simulink model "ex_4_PID"  (R2018a)
settings: Solver=VariableStepAuto  StartTime=0.0  StopTime=20  RelTol=1e-3
values from neighbouring files (symbols this model uses):
  b = 1    [EX4_MATHLAB_SCRIPT.m]
  D = 5    [EX4_MATHLAB_SCRIPT.m]
  den1 = [J*Ra,Kb*Km,K*Km]    [EX4_MATHLAB_SCRIPT.m]
  den2 = [J*Ra,Kb*Km,K*Km]    [EX4_MATHLAB_SCRIPT.m]
  I = 10    [EX4_MATHLAB_SCRIPT.m]
  J = 0.1    [EX4_MATHLAB_SCRIPT.m]
  Kb = 1    [EX4_MATHLAB_SCRIPT.m]
  Km = 0.1    [EX4_MATHLAB_SCRIPT.m]
  La = 1    [EX4_MATHLAB_SCRIPT.m]
  n = 10    [EX4_MATHLAB_SCRIPT.m]
  num1 = [K*Km]    [EX4_MATHLAB_SCRIPT.m]
  num2 = [Km,0]    [EX4_MATHLAB_SCRIPT.m]
  P = 50    [EX4_MATHLAB_SCRIPT.m]
  Ra = 20    [EX4_MATHLAB_SCRIPT.m]
libraries: simulink x2
settings Model: Creator=k2202936  LastModifiedBy=k2202936

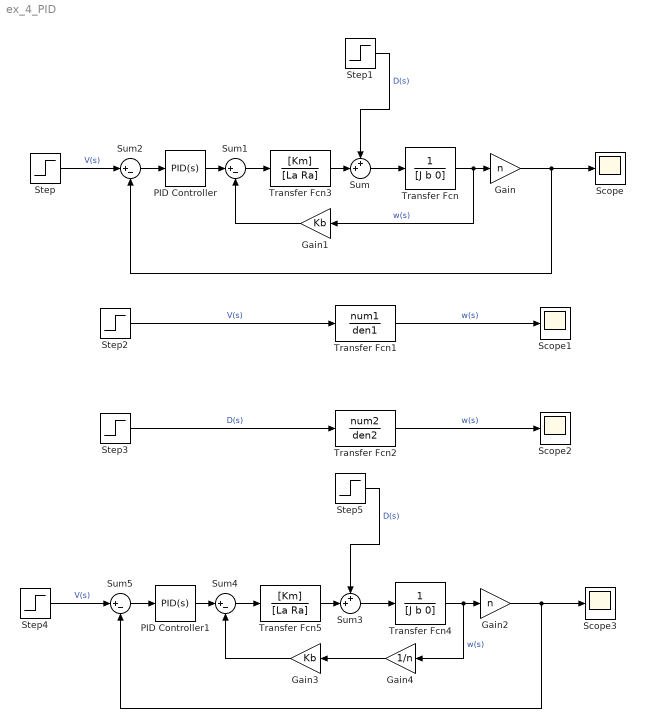
== system ex_4_PID ==
  Gain : Gain  Gain=n
  Gain1 : Gain  Gain=Kb
  Gain2 : Gain  Gain=n
  Gain3 : Gain  Gain=Kb
  Gain4 : Gain  Gain=1/n
  PID Controller : simulink/Continuous/PID Controller  Controller=PID  TimeDomain=Continuous-time  SampleTime=-1  IntegratorMethod=Forward Euler  FilterMethod=Forward Euler  Form=Parallel  UseFilter=on  ControllerParametersSource=internal  P=P  I=I  D=D  N=100  InitialConditionSource=internal  InitialConditionForIntegrator=0  InitialConditionForFilter=0  ExternalReset=none  LimitOutput=off  UpperSaturationLimit=inf  LowerSaturationLimit=-inf  LinearizeAsGain=on  AntiWindupMode=none  Kb=1  TrackingMode=off  Kt=1  PParamMin=[]  PParamMax=[]  IParamMin=[]  IParamMax=[]  DParamMin=[]  DParamMax=[]  NParamMin=[]  NParamMax=[]  KbParamMin=[]  KbParamMax=[]  KtParamMin=[]  KtParamMax=[]  POutMin=[]  POutMax=[]  IOutMin=[]  IOutMax=[]  DOutMin=[]  DOutMax=[]  NOutMin=[]  NOutMax=[]  KbOutMin=[]  KbOutMax=[]  KtOutMin=[]  KtOutMax=[]  IntegratorOutMin=[]  IntegratorOutMax=[]  FilterOutMin=[]  FilterOutMax=[]  SumOutMin=[]  SumOutMax=[]  SumI1OutMin=[]  SumI1OutMax=[]  SumI2OutMin=[]  SumI2OutMax=[]  SumI3OutMin=[]  SumI3OutMax=[]  SumDOutMin=[]  SumDOutMax=[]  SaturationOutMin=[]  SaturationOutMax=[]  IntegratorContinuousStateAttributes=''  IntegratorStateMustResolveToSignalObject=off  IntegratorRTWStateStorageClass=Auto  FilterContinuousStateAttributes=''  FilterStateMustResolveToSignalObject=off  FilterRTWStateStorageClass=Auto  DifferentiatorICPrevScaledInput=0  DifferentiatorOutMin=[]  DifferentiatorOutMax=[]  FilterDiffOutCoefMin=[]  FilterDiffOutCoefMax=[]  SumDenOutMin=[]  SumDenOutMax=[]  SumNumOutMin=[]  SumNumOutMax=[]  ReciprocalOutMin=[]  ReciprocalOutMax=[]  DivideOutMin=[]  DivideOutMax=[]  TunerSelectOption=Transfer Function Based (PID Tuner App)
  PID Controller1 : simulink/Continuous/PID Controller  Controller=PID  TimeDomain=Continuous-time  SampleTime=-1  IntegratorMethod=Forward Euler  FilterMethod=Forward Euler  Form=Parallel  UseFilter=on  ControllerParametersSource=internal  P=P  I=I  D=D  N=100  InitialConditionSource=internal  InitialConditionForIntegrator=0  InitialConditionForFilter=0  ExternalReset=none  LimitOutput=off  UpperSaturationLimit=inf  LowerSaturationLimit=-inf  LinearizeAsGain=on  AntiWindupMode=none  Kb=1  TrackingMode=off  Kt=1  PParamMin=[]  PParamMax=[]  IParamMin=[]  IParamMax=[]  DParamMin=[]  DParamMax=[]  NParamMin=[]  NParamMax=[]  KbParamMin=[]  KbParamMax=[]  KtParamMin=[]  KtParamMax=[]  POutMin=[]  POutMax=[]  IOutMin=[]  IOutMax=[]  DOutMin=[]  DOutMax=[]  NOutMin=[]  NOutMax=[]  KbOutMin=[]  KbOutMax=[]  KtOutMin=[]  KtOutMax=[]  IntegratorOutMin=[]  IntegratorOutMax=[]  FilterOutMin=[]  FilterOutMax=[]  SumOutMin=[]  SumOutMax=[]  SumI1OutMin=[]  SumI1OutMax=[]  SumI2OutMin=[]  SumI2OutMax=[]  SumI3OutMin=[]  SumI3OutMax=[]  SumDOutMin=[]  SumDOutMax=[]  SaturationOutMin=[]  SaturationOutMax=[]  IntegratorContinuousStateAttributes=''  IntegratorStateMustResolveToSignalObject=off  IntegratorRTWStateStorageClass=Auto  FilterContinuousStateAttributes=''  FilterStateMustResolveToSignalObject=off  FilterRTWStateStorageClass=Auto  DifferentiatorICPrevScaledInput=0  DifferentiatorOutMin=[]  DifferentiatorOutMax=[]  FilterDiffOutCoefMin=[]  FilterDiffOutCoefMax=[]  SumDenOutMin=[]  SumDenOutMax=[]  SumNumOutMin=[]  SumNumOutMax=[]  ReciprocalOutMin=[]  ReciprocalOutMax=[]  DivideOutMin=[]  DivideOutMax=[]  TunerSelectOption=Transfer Function Based (PID Tuner App)
  Scope{,1..3} (4 alike) : Scope
  Step{,2..3,5} (4 alike) : Step  Time=0  SampleTime=0
  Step1 : Step  Time=0  After=0  SampleTime=0
  Step4 : Step  Time=0  After=0  SampleTime=0
  Sum : Sum  Inputs=++|
  Sum{1..2,4..5} (4 alike) : Sum  Inputs=|+-
  Sum3 : Sum  Inputs=++|
  Transfer Fcn : TransferFcn  Denominator=[J b 0]
  Transfer Fcn1 : TransferFcn  Numerator=num1  Denominator=den1
  Transfer Fcn2 : TransferFcn  Numerator=num2  Denominator=den2
  Transfer Fcn3 : TransferFcn  Numerator=[Km]  Denominator=[La Ra]
  Transfer Fcn4 : TransferFcn  Denominator=[J b 0]
  Transfer Fcn5 : TransferFcn  Numerator=[Km]  Denominator=[La Ra]
  wires:
  Step3/1 -> Transfer Fcn2/1  "D(s)"
  Step2/1 -> Transfer Fcn1/1  "V(s)"
  Transfer Fcn2/1 -> Scope2/1  "w(s)"
  Transfer Fcn1/1 -> Scope1/1  "w(s)"
  Sum/1 -> Transfer Fcn/1
  Sum2/1 -> PID Controller/1
  Transfer Fcn/1 -> Gain1/1, Gain/1  "w(s)"
  Sum1/1 -> Transfer Fcn3/1
  Step/1 -> Sum2/1  "V(s)"
  Transfer Fcn3/1 -> Sum/2
  Step1/1 -> Sum/1  "D(s)"
  PID Controller/1 -> Sum1/1
  Gain1/1 -> Sum1/2
  Gain/1 -> Sum2/2, Scope/1
  Sum4/1 -> Transfer Fcn5/1
  Gain2/1 -> Sum5/2, Scope3/1
  Transfer Fcn5/1 -> Sum3/2
  Sum5/1 -> PID Controller1/1
  PID Controller1/1 -> Sum4/1
  Step4/1 -> Sum5/1  "V(s)"
  Sum3/1 -> Transfer Fcn4/1
  Gain3/1 -> Sum4/2
  Transfer Fcn4/1 -> Gain4/1, Gain2/1  "w(s)"
  Step5/1 -> Sum3/1  "D(s)"
  Gain4/1 -> Gain3/1
